simulink model "Chassis"  (R2013a)
settings: Solver=ode45  StartTime=0.0  StopTime=10.0  RelTol=1e-3
model workspace: external: MAT-File Vehicle\Chassis\Data\Chassis.mat (data not in the file)
undefined symbols (not defined in the file): CdA, d0, g, m, v0
settings Model: Creator=Nathan  LastModifiedBy=Nathan
settings OptimizationCC: InlineParams=on

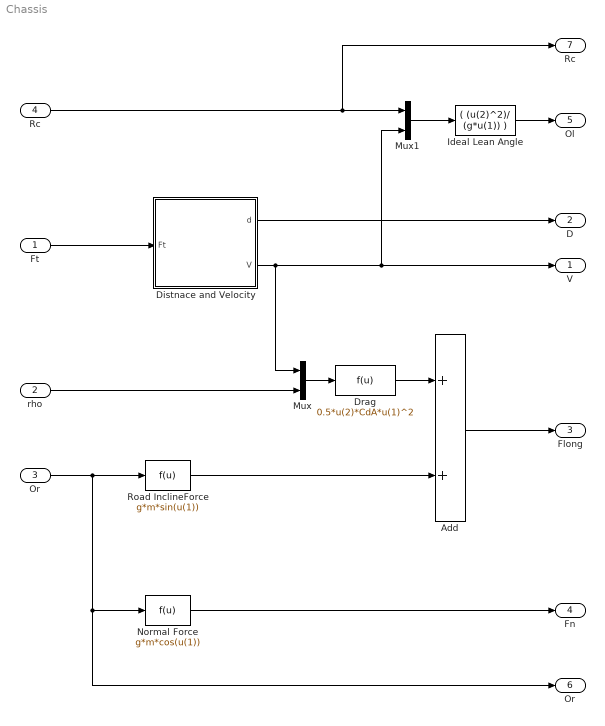
== system Chassis ==
  Ft : Inport
  rho : Inport  Port=2
  Or : Inport  Port=3
  Rc : Inport  Port=4
  Add : Sum
  Distnace and Velocity : Subsystem
  Drag : Fcn  Expr=0.5*u(2)*CdA*u(1)^2
  Ideal Lean Angle : Fcn  Expr=( (u(2)^2)/ (g*u(1)) )
  Mux : Mux  Inputs=2
  Mux1 : Mux  Inputs=2
  Normal Force : Fcn  Expr=g*m*cos(u(1))
  Road InclineForce : Fcn  Expr=g*m*sin(u(1))
  V : Outport
  D : Outport  Port=2
  Flong : Outport  Port=3
  Fn : Outport  Port=4
  Ol : Outport  Port=5
  "Or " : Outport  Port=6
  "Rc " : Outport  Port=7
  wires:
  Distnace and Velocity/2(V) -> Mux/1, Mux1/2, V/1
  Distnace and Velocity/1(d) -> D/1
  Mux/1 -> Drag/1
  rho/1 -> Mux/2
  Or/1 -> "Or "/1, Normal Force/1, Road InclineForce/1
  Drag/1 -> Add/1
  Normal Force/1 -> Fn/1
  Mux1/1 -> Ideal Lean Angle/1
  Rc/1 -> "Rc "/1, Mux1/1
  Ideal Lean Angle/1 -> Ol/1
  Ft/1 -> Distnace and Velocity/1(Ft)
  Road InclineForce/1 -> Add/2
  Add/1 -> Flong/1

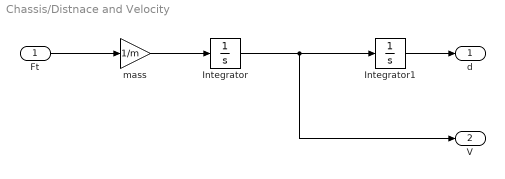
== system Chassis/Distnace and Velocity ==
  Ft : Inport
  Integrator : Integrator  InitialCondition=v0
  Integrator1 : Integrator  InitialCondition=d0
  mass : Gain  Gain=1/m
  d : Outport
  V : Outport  Port=2
  wires:
  Ft/1 -> mass/1
  mass/1 -> Integrator/1
  Integrator/1 -> Integrator1/1, V/1
  Integrator1/1 -> d/1
